simulink model "test_newfft_fun"  (Simulink 6.2)
settings: Solver=ode45  StartTime=0.0  StopTime=850  RelTol=1e-3
libraries: xbsIndex_r3 x554, simulink x1
(part 5 of 9)

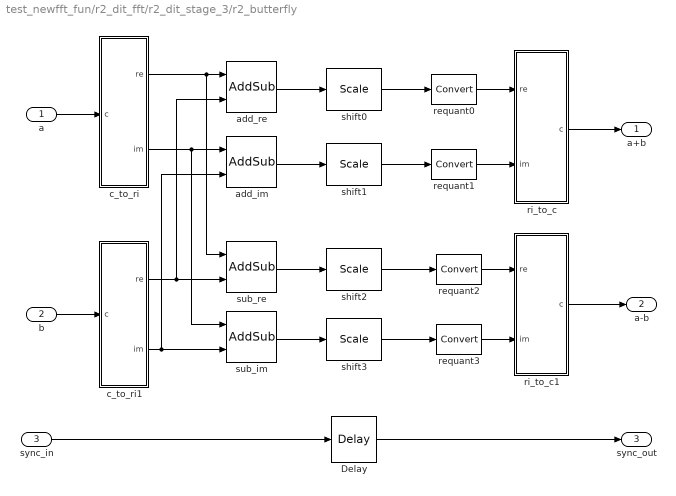
== system test_newfft_fun/r2_dit_fft/r2_dit_stage_3/r2_butterfly ==
  a : Inport  Port=1  LatchInput=off
  b : Inport  Port=2  LatchInput=off
  sync_in : Inport  Port=3  LatchInput=off
  Delay : xbsIndex_r3/Delay  latency=1  reg_retiming=off  explicit_period=off  period=1  en=off  accept_only_valid=off  init_zero=on  dbl_ovrd=off  show_param=off
      settings: xl_area=[0, 0, 0, 0, 0, 0, 0]
  add_im : xbsIndex_r3/AddSub  mode=Addition  precision=Full  arith_type=Unsigned  n_bits=8  bin_pt=2  quantization=Truncate  overflow=Wrap  latency=1  explicit_period=off  period=1  use_carryin=off  use_carryout=off  en=off  dbl_ovrd=off  show_param=on  use_core=on  pipeline=on  use_rpm=on  gen_core=off
      settings: xl_area=[0, 0, 0, 0, 0, 0, 0]
  add_re : xbsIndex_r3/AddSub  mode=Addition  precision=Full  arith_type=Unsigned  n_bits=8  bin_pt=2  quantization=Truncate  overflow=Wrap  latency=1  explicit_period=off  period=1  use_carryin=off  use_carryout=off  en=off  dbl_ovrd=off  show_param=on  use_core=on  pipeline=on  use_rpm=on  gen_core=off
      settings: xl_area=[0, 0, 0, 0, 0, 0, 0]
  c_to_ri : Subsystem  mask(Complex to Real-Imag){n_bits=10, bin_pt=0}
      mask prompts: n_bits "Bit Width"; bin_pt "Binary Point"
      mask help: Outputs real and imaginary components of a complex input.
      settings: AttributesFormatString=10_0 r/i
      mask Help:
      | <pre>
      | Description::
      | 
      | Outputs real and imaginary components of a complex input.
      | Useful for simplifying interconnects.
      | See also: Real-Imag to Complex (ri_to_c)
      | 
      | Mask Parameters::
      | 
      | Bit Width (n_bits): Specifies the width of the real/imaginary components.
      | Assumed equal for both components.
      | 
      | Binary Point (bin_pt): Specifies the binary point location in the real/imaginary components.
      | Assumed equal for both components.
      | </pre>
  c_to_ri1 : Subsystem  mask(Complex to Real-Imag){n_bits=10, bin_pt=0}
      mask prompts: n_bits "Bit Width"; bin_pt "Binary Point"
      mask help: Outputs real and imaginary components of a complex input.
      settings: AttributesFormatString=10_0 r/i
      mask Help:
      | <pre>
      | Description::
      | 
      | Outputs real and imaginary components of a complex input.
      | Useful for simplifying interconnects.
      | See also: Real-Imag to Complex (ri_to_c)
      | 
      | Mask Parameters::
      | 
      | Bit Width (n_bits): Specifies the width of the real/imaginary components.
      | Assumed equal for both components.
      | 
      | Binary Point (bin_pt): Specifies the binary point location in the real/imaginary components.
      | Assumed equal for both components.
      | </pre>
  requant{0..3} (4 alike) : xbsIndex_r3/Convert  arith_type="Signed  (2's comp)"  n_bits=11  bin_pt=0  quantization=Truncate  overflow=Wrap  latency=0  explicit_period=off  period=1  dbl_ovrd=off  show_param=on  inserted_by_tool=off  pipeline=on
      settings: xl_area=[0, 0, 0, 0, 0, 0, 0]
  ri_to_c : Subsystem
      mask Type: Real-Imag to Complex
      mask Description: Concatenates real and imaginary inputs into a complex output.
      mask Help:
      | <pre>
      | Description::
      | 
      | Concatenates a real and imaginary input into a complex output.
      | Useful for simplifying interconnects.
      | See also: Complex to Real-Imag (c_to_ri)
      | 
      | Mask Parameters::
      | 
      | (N/A)
      | </pre>
  ri_to_c1 : Subsystem
      mask Type: Real-Imag to Complex
      mask Description: Concatenates real and imaginary inputs into a complex output.
      mask Help:
      | <pre>
      | Description::
      | 
      | Concatenates a real and imaginary input into a complex output.
      | Useful for simplifying interconnects.
      | See also: Complex to Real-Imag (c_to_ri)
      | 
      | Mask Parameters::
      | 
      | (N/A)
      | </pre>
  shift{0..3} (4 alike) : xbsIndex_r3/Scale  scale_factor=0  explicit_period=off  period=1  dbl_ovrd=off
  sub_im : xbsIndex_r3/AddSub  mode=Subtraction  precision=Full  arith_type=Unsigned  n_bits=8  bin_pt=2  quantization=Truncate  overflow=Wrap  latency=1  explicit_period=off  period=1  use_carryin=off  use_carryout=off  en=off  dbl_ovrd=off  show_param=on  use_core=on  pipeline=on  use_rpm=on  gen_core=off
      settings: xl_area=[0, 0, 0, 0, 0, 0, 0]
  sub_re : xbsIndex_r3/AddSub  mode=Subtraction  precision=Full  arith_type=Unsigned  n_bits=8  bin_pt=2  quantization=Truncate  overflow=Wrap  latency=1  explicit_period=off  period=1  use_carryin=off  use_carryout=off  en=off  dbl_ovrd=off  show_param=on  use_core=on  pipeline=on  use_rpm=on  gen_core=off
      settings: xl_area=[0, 0, 0, 0, 0, 0, 0]
  a+b : Outport
  a-b : Outport  Port=2
  sync_out : Outport  Port=3
  wires:
  shift3/1 -> requant3/1
  sub_im/1 -> shift3/1
  shift2/1 -> requant2/1
  sub_re/1 -> shift2/1
  shift1/1 -> requant1/1
  shift0/1 -> requant0/1
  requant3/1 -> ri_to_c1/2(im)
  requant2/1 -> ri_to_c1/1(re)
  requant1/1 -> ri_to_c/2(im)
  requant0/1 -> ri_to_c/1(re)
  Delay/1 -> sync_out/1
  sync_in/1 -> Delay/1
  ri_to_c1/1(c) -> a-b/1
  ri_to_c/1(c) -> a+b/1
  add_im/1 -> shift1/1
  add_re/1 -> shift0/1
  a/1 -> c_to_ri/1(c)
  c_to_ri/2(im) -> sub_im/1, add_im/1
  c_to_ri/1(re) -> sub_re/1, add_re/1
  c_to_ri1/2(im) -> add_im/2, sub_im/2
  c_to_ri1/1(re) -> add_re/2, sub_re/2
  b/1 -> c_to_ri1/1(c)

== system test_newfft_fun/r2_dit_fft/r2_dit_stage_3/r2_twiddle ==
  a_in : Inport  Port=1  LatchInput=off
  b : Inport  Port=2  LatchInput=off
  sync_in : Inport  Port=3  LatchInput=off
  Delay1 : xbsIndex_r3/Delay  latency=1  reg_retiming=off  explicit_period=off  period=1  en=off  accept_only_valid=off  init_zero=on  dbl_ovrd=off  show_param=off
      settings: xl_area=[0, 0, 0, 0, 0, 0, 0]
  Delay2 : xbsIndex_r3/Delay  latency=1  reg_retiming=off  explicit_period=off  period=1  en=off  accept_only_valid=off  init_zero=on  dbl_ovrd=off  show_param=off
      settings: xl_area=[0, 0, 0, 0, 0, 0, 0]
  Delay3 : xbsIndex_r3/Delay  latency=1  reg_retiming=off  explicit_period=off  period=1  en=off  accept_only_valid=off  init_zero=on  dbl_ovrd=off  show_param=off
      settings: xl_area=[0, 0, 0, 0, 0, 0, 0]
  cmpy1 : Subsystem  mask(Complex Multiplier (4 real multipliers)){n_bits_b=10, bin_pt_b=9, n_bits_w=8, bin_pt_w=6, n_bits_bw=10, bin_pt_bw=9, quantization=Round  (unbiased: Even Values), overflow=Wrap, mult_latency=3, add_latency=1}
      mask prompts: n_bits_b "Number of Bits B"; bin_pt_b "Binary Point B"; n_bits_w "Number of Bits W"; bin_pt_w "Binary Point W"; n_bits_bw "Number of Bits BW"; bin_pt_bw "Binary Point BW"; mult_latency "Multiplier Latency"; add_latency "Adder Latency"
      mask help: This block multiplies two complex numbers using 4 real multipliers and 2 real adders. Pass-through paths are provided for another complex number and a sync signal. These pass through paths provide delay that matches the latency of the complex multiply operation.
      settings: AttributesFormatString=|
      | 10_9 * 8_6 ==> 10_9
      | round even, wrap
      | 3 mults
      mask Help:
      | <pre>
      | Description::
      | 
      | This block multiplies two complex numbers using 4 real multipliers and 2 real adders.
      | Pass-through paths are provided for another complex number and a sync signal.
      | These paths provide delay that matches the latency of the complex multiply operation.
      | 
      | a_in is passed through to a_out.
      | b and w complex inputs are multiplied and their product appears on the bw output.
      | sync_in is passed through to sync_out.
      | 
      | Mask Parameters::
      | 
      | Number of Bits B (n_bits_b): Specifies the width of the real/imaginary
      | components of input b.  Assumed equal for both components.
      | 
      | Binary Point B (bin_pt_b): Specifies the binary point point position of the
      | real/imaginary components of input b.  Assumed equal for both components.
      | 
      | Number of Bits W (n_bits_w): Specifies the width of the real/imaginary
      | components of input w.  Assumed equal for both components.
      | 
      | Binary Point W (bin_pt_w): Specifies the binary point point position of the
      | real/imaginary components of input w.  Assumed equal for both components.
      | 
      | Number of Bits BW (n_bits_bw): Specifies the width of the real/imaginary
      | components of output bw.  Assumed equal for both components.
      | 
      | Binary Point BW (bin_pt_bw): Specifies the binary point point position of the
      | real/imaginary components of output bw.  Assumed equal for both components.
      | 
      | Quantization (quantization): Specifies quantization handling.
      | 
      | Overflow (overflow): Specifies overflow handling.
      | 
      | Multiplier Latency (mult_latency): Latency to use for the underlying real multipliers.
      | 
      | Adder Latency (add_latency): Latency to use for the underlying real adders.
      | </pre>
      mask StyleString: edit,edit,edit,edit,edit,edit,popup(Truncate|Round  (unbiased: +/- Inf)|Round  (unbiased: Even Values)),popup(Wrap|Saturate|Error),edit,edit
  twiddle_gen1 : Subsystem  mask(Radix-R Twiddle Coefficient Generator (complex storage)){n_stages=8, radix=2, cur_stage=3, branch=1, decimation=Time, n_bits_w=8, bin_pt_w=6, use_bram=off}
      mask prompts: n_stages "Total Stages"; cur_stage "Current Stage"; decimation "Decimation Mode"; n_bits_w "Number of Bits"; bin_pt_w "Binary Point"; use_bram "Use BRAM"
      mask help: A radix-R twiddle coefficient generator using complex storage. Generates twiddle factors for Decimation in Time (i.e. twiddles before butterflies) or Decimation in Frequency (i.e. twiddles after butterflies) Fast Fourier Transforms of arbitrary-but-fixed radix. Radix must be a power of 2. Regardless of the decimation mode, the FFT is assumed to have inputs in normal order and outputs in bit-reversed order.
      settings: AttributesFormatString=|
      | depth 4
      | twiddle dist
      mask Help:
      | <pre>
      | Description::
      | 
      | A radix-R twiddle coefficient generator using complex storage.
      | 
      | Generates twiddle factors for Decimation in Time (i.e. twiddles before butterflies)
      | or Decimation in Frequency (i.e. twiddles after butterflies) Fast Fourier Transforms
      | of arbitrary-but-fixed radix.  Radix must be a power of 2.
      | 
      | Regardless of the decimation mode, the FFT is assumed to have inputs normally
      | ordered and outputs in bit-reversed order.
      | 
      | Complex storage means that the real and imaginary components are stored in
      | the same memory element.  This is generally fine, but if the combined width of
      | the real and imaginary components is greater than 18 and BRAM is being used
      | for the underlying storage, then the multiplier(s) adjacent to the BRAM(s) will
      | not be usable.  If that is a problem for your design, consider using the
      | "Radix-R Twiddle Coefficient Generator (real/imag storage)" block.
      | 
      | Mask Parameters::
      | 
      | Total Stages (n_stages):  The number of total stages in the FFT.
      | 
      | Radix (radix): The radix of the FFT.  The FFT will have radix^n_stages points.
      | 
      | Current Stage (cur_stage):  The number of the current stage for which this block should
      | generate twiddle coefficients.  Valid values are 3 through n_stages, inclusive.  Note that
      | stages are counted from 1 to n_stages for DIT (i.e. cur_stage==1 for the first stage) and
      | n_stages to 1 for DIF (i.e. cur_stage==1 for the last stage).
      | 
      | Branch (branch): The butterfly branch associated with this twiddle generator.
      | Valid values are 1 through radix-1, inclusive.
      | 
      | Decimation Mode (decimation): The decimation mode of the FFT.
      | 
      | Number of Bits (n_bits_w): Specifies the width of the real/imaginary components.
      | Assumed equal for both components.  This block outputs UFix_(2*n_bits_w)_0.
      | 
      | Use BRAM (use_bram): Check this checkbox to store twiddle coefficients in BRAM.
      | If unchecked, the coefficients will be sored in distributed memory (i.e. slices).
      | </pre>
      mask StyleString: edit,edit,edit,edit,popup(Time|Frequency),edit,edit,checkbox
  a_out : Outport
  bw : Outport  Port=2
  sync_out : Outport  Port=3
  wires:
  Delay3/1 -> cmpy1/4(sync_in)
  cmpy1/3(sync_out) -> sync_out/1
  twiddle_gen1/1(w) -> cmpy1/3(w)
  cmpy1/2(bw) -> bw/1
  Delay1/1 -> cmpy1/2(b)
  cmpy1/1(a_out) -> a_out/1
  Delay2/1 -> cmpy1/1(a_in)
  a_in/1 -> Delay2/1
  b/1 -> Delay1/1
  sync_in/1 -> Delay3/1, twiddle_gen1/1(sync_in)

== system test_newfft_fun/r2_dit_fft/r2_dit_stage_4/biplex_commutator ==
  AloAhi : Inport  Port=1  LatchInput=off
  BloBhi : Inport  Port=2  LatchInput=off
  sync_in : Inport  Port=3  LatchInput=off
  Counter : xbsIndex_r3/Counter  cnt_type=Free Running  n_bits=5  bin_pt=0  arith_type=Unsigned  start_count=0  cnt_to=Inf  cnt_by_val=1  operation=Up  explicit_period=off  period=1  load_pin=off  rst=on  en=off  dbl_ovrd=off  show_param=off  use_rpm=on  gen_core=off
      settings: xl_area=[0, 0, 0, 0, 0, 0, 0]
  Delay : xbsIndex_r3/Delay  latency=17  reg_retiming=off  explicit_period=off  period=1  en=off  accept_only_valid=off  init_zero=on  dbl_ovrd=off  show_param=off
      settings: xl_area=[0, 0, 0, 0, 0, 0, 0]
  Mux : xbsIndex_r3/Mux  inputs=2  precision=Full  arith_type="Signed  (2's comp)"  n_bits=8  bin_pt=2  quantization=Truncate  overflow=Wrap  latency=1  explicit_period=off  period=1  en=off  dbl_ovrd=off  show_param=off  mux_type=off  use_rpm=off  gen_core=off
      settings: xl_area=[0, 0, 0, 0, 0, 0, 0]
  Mux1 : xbsIndex_r3/Mux  inputs=2  precision=Full  arith_type="Signed  (2's comp)"  n_bits=8  bin_pt=2  quantization=Truncate  overflow=Wrap  latency=1  explicit_period=off  period=1  en=off  dbl_ovrd=off  show_param=on  mux_type=off  use_rpm=off  gen_core=off
      settings: xl_area=[0, 0, 0, 0, 0, 0, 0]
  delay_b : Subsystem  mask(SLR16 Delay){delay_depth=16}
      mask prompts: delay_depth "Delay Depth"
      mask help: A delay block that uses SLR16 elements for its storage.
      settings: AttributesFormatString=slr depth = 16
      mask Help:
      | <pre>
      | Description::
      | 
      | A delay block that uses SLR16 elements for its storage.
      | 
      | Mask Parameters::
      | 
      | Delay Depth (delay_depth): The length of the delay.
      | </pre>
  delay_lo : Subsystem  mask(SLR16 Delay){delay_depth=16}
      mask prompts: delay_depth "Delay Depth"
      mask help: A delay block that uses SLR16 elements for its storage.
      settings: AttributesFormatString=slr depth = 16
      mask Help:
      | <pre>
      | Description::
      | 
      | A delay block that uses SLR16 elements for its storage.
      | 
      | Mask Parameters::
      | 
      | Delay Depth (delay_depth): The length of the delay.
      | </pre>
  top_bit : xbsIndex_r3/Slice  mode=Upper Bit Location + Width  nbits=1  bit1=0  base1=MSB of Input  bit0=0  base0=LSB of Input  boolean_output=off  explicit_period=off  period=1  dbl_ovrd=off
  AloBlo : Outport
  AhiBhi : Outport  Port=2
  sync_out : Outport  Port=3
  wires:
  Delay/1 -> sync_out/1
  delay_lo/1(out) -> AloBlo/1
  Mux/1 -> delay_lo/1(in)
  delay_b/1(out) -> Mux/3, Mux1/2
  BloBhi/1 -> delay_b/1(in)
  Mux1/1 -> AhiBhi/1
  AloAhi/1 -> Mux1/3, Mux/2
  top_bit/1 -> Mux/1, Mux1/1
  Counter/1 -> top_bit/1
  sync_in/1 -> Delay/1, Counter/1

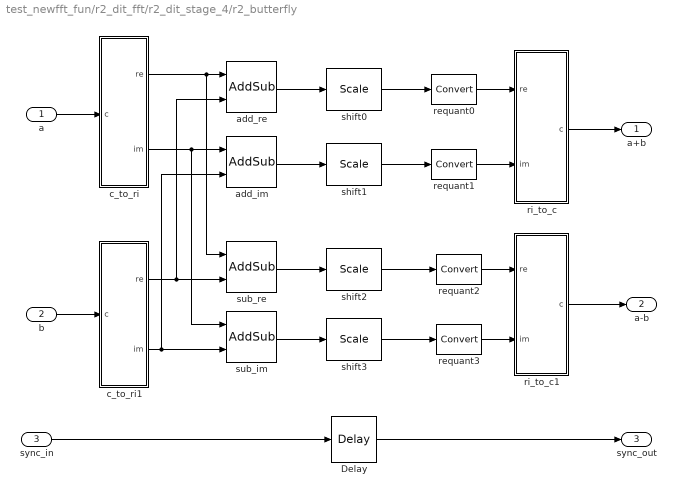
== system test_newfft_fun/r2_dit_fft/r2_dit_stage_4/r2_butterfly ==
  a : Inport  Port=1  LatchInput=off
  b : Inport  Port=2  LatchInput=off
  sync_in : Inport  Port=3  LatchInput=off
  Delay : xbsIndex_r3/Delay  latency=1  reg_retiming=off  explicit_period=off  period=1  en=off  accept_only_valid=off  init_zero=on  dbl_ovrd=off  show_param=off
      settings: xl_area=[0, 0, 0, 0, 0, 0, 0]
  add_im : xbsIndex_r3/AddSub  mode=Addition  precision=Full  arith_type=Unsigned  n_bits=8  bin_pt=2  quantization=Truncate  overflow=Wrap  latency=1  explicit_period=off  period=1  use_carryin=off  use_carryout=off  en=off  dbl_ovrd=off  show_param=on  use_core=on  pipeline=on  use_rpm=on  gen_core=off
      settings: xl_area=[0, 0, 0, 0, 0, 0, 0]
  add_re : xbsIndex_r3/AddSub  mode=Addition  precision=Full  arith_type=Unsigned  n_bits=8  bin_pt=2  quantization=Truncate  overflow=Wrap  latency=1  explicit_period=off  period=1  use_carryin=off  use_carryout=off  en=off  dbl_ovrd=off  show_param=on  use_core=on  pipeline=on  use_rpm=on  gen_core=off
      settings: xl_area=[0, 0, 0, 0, 0, 0, 0]
  c_to_ri : Subsystem  mask(Complex to Real-Imag){n_bits=11, bin_pt=0}
      mask prompts: n_bits "Bit Width"; bin_pt "Binary Point"
      mask help: Outputs real and imaginary components of a complex input.
      settings: AttributesFormatString=11_0 r/i
      mask Help:
      | <pre>
      | Description::
      | 
      | Outputs real and imaginary components of a complex input.
      | Useful for simplifying interconnects.
      | See also: Real-Imag to Complex (ri_to_c)
      | 
      | Mask Parameters::
      | 
      | Bit Width (n_bits): Specifies the width of the real/imaginary components.
      | Assumed equal for both components.
      | 
      | Binary Point (bin_pt): Specifies the binary point location in the real/imaginary components.
      | Assumed equal for both components.
      | </pre>
  c_to_ri1 : Subsystem  mask(Complex to Real-Imag){n_bits=11, bin_pt=0}
      mask prompts: n_bits "Bit Width"; bin_pt "Binary Point"
      mask help: Outputs real and imaginary components of a complex input.
      settings: AttributesFormatString=11_0 r/i
      mask Help:
      | <pre>
      | Description::
      | 
      | Outputs real and imaginary components of a complex input.
      | Useful for simplifying interconnects.
      | See also: Real-Imag to Complex (ri_to_c)
      | 
      | Mask Parameters::
      | 
      | Bit Width (n_bits): Specifies the width of the real/imaginary components.
      | Assumed equal for both components.
      | 
      | Binary Point (bin_pt): Specifies the binary point location in the real/imaginary components.
      | Assumed equal for both components.
      | </pre>
  requant{0..3} (4 alike) : xbsIndex_r3/Convert  arith_type="Signed  (2's comp)"  n_bits=12  bin_pt=0  quantization=Truncate  overflow=Wrap  latency=0  explicit_period=off  period=1  dbl_ovrd=off  show_param=on  inserted_by_tool=off  pipeline=on
      settings: xl_area=[0, 0, 0, 0, 0, 0, 0]
  ri_to_c : Subsystem
      mask Type: Real-Imag to Complex
      mask Description: Concatenates real and imaginary inputs into a complex output.
      mask Help:
      | <pre>
      | Description::
      | 
      | Concatenates a real and imaginary input into a complex output.
      | Useful for simplifying interconnects.
      | See also: Complex to Real-Imag (c_to_ri)
      | 
      | Mask Parameters::
      | 
      | (N/A)
      | </pre>
  ri_to_c1 : Subsystem
      mask Type: Real-Imag to Complex
      mask Description: Concatenates real and imaginary inputs into a complex output.
      mask Help:
      | <pre>
      | Description::
      | 
      | Concatenates a real and imaginary input into a complex output.
      | Useful for simplifying interconnects.
      | See also: Complex to Real-Imag (c_to_ri)
      | 
      | Mask Parameters::
      | 
      | (N/A)
      | </pre>
  shift{0..3} (4 alike) : xbsIndex_r3/Scale  scale_factor=0  explicit_period=off  period=1  dbl_ovrd=off
  sub_im : xbsIndex_r3/AddSub  mode=Subtraction  precision=Full  arith_type=Unsigned  n_bits=8  bin_pt=2  quantization=Truncate  overflow=Wrap  latency=1  explicit_period=off  period=1  use_carryin=off  use_carryout=off  en=off  dbl_ovrd=off  show_param=on  use_core=on  pipeline=on  use_rpm=on  gen_core=off
      settings: xl_area=[0, 0, 0, 0, 0, 0, 0]
  sub_re : xbsIndex_r3/AddSub  mode=Subtraction  precision=Full  arith_type=Unsigned  n_bits=8  bin_pt=2  quantization=Truncate  overflow=Wrap  latency=1  explicit_period=off  period=1  use_carryin=off  use_carryout=off  en=off  dbl_ovrd=off  show_param=on  use_core=on  pipeline=on  use_rpm=on  gen_core=off
      settings: xl_area=[0, 0, 0, 0, 0, 0, 0]
  a+b : Outport
  a-b : Outport  Port=2
  sync_out : Outport  Port=3
  wires:
  shift3/1 -> requant3/1
  sub_im/1 -> shift3/1
  shift2/1 -> requant2/1
  sub_re/1 -> shift2/1
  shift1/1 -> requant1/1
  shift0/1 -> requant0/1
  requant3/1 -> ri_to_c1/2(im)
  requant2/1 -> ri_to_c1/1(re)
  requant1/1 -> ri_to_c/2(im)
  requant0/1 -> ri_to_c/1(re)
  Delay/1 -> sync_out/1
  sync_in/1 -> Delay/1
  ri_to_c1/1(c) -> a-b/1
  ri_to_c/1(c) -> a+b/1
  add_im/1 -> shift1/1
  add_re/1 -> shift0/1
  a/1 -> c_to_ri/1(c)
  c_to_ri/2(im) -> sub_im/1, add_im/1
  c_to_ri/1(re) -> sub_re/1, add_re/1
  c_to_ri1/2(im) -> add_im/2, sub_im/2
  c_to_ri1/1(re) -> add_re/2, sub_re/2
  b/1 -> c_to_ri1/1(c)

== system test_newfft_fun/r2_dit_fft/r2_dit_stage_4/r2_twiddle ==
  a_in : Inport  Port=1  LatchInput=off
  b : Inport  Port=2  LatchInput=off
  sync_in : Inport  Port=3  LatchInput=off
  Delay1 : xbsIndex_r3/Delay  latency=1  reg_retiming=off  explicit_period=off  period=1  en=off  accept_only_valid=off  init_zero=on  dbl_ovrd=off  show_param=off
      settings: xl_area=[0, 0, 0, 0, 0, 0, 0]
  Delay2 : xbsIndex_r3/Delay  latency=1  reg_retiming=off  explicit_period=off  period=1  en=off  accept_only_valid=off  init_zero=on  dbl_ovrd=off  show_param=off
      settings: xl_area=[0, 0, 0, 0, 0, 0, 0]
  Delay3 : xbsIndex_r3/Delay  latency=1  reg_retiming=off  explicit_period=off  period=1  en=off  accept_only_valid=off  init_zero=on  dbl_ovrd=off  show_param=off
      settings: xl_area=[0, 0, 0, 0, 0, 0, 0]
  cmpy1 : Subsystem  mask(Complex Multiplier (4 real multipliers)){n_bits_b=11, bin_pt_b=10, n_bits_w=8, bin_pt_w=6, n_bits_bw=11, bin_pt_bw=10, quantization=Round  (unbiased: Even Values), overflow=Wrap, mult_latency=3, add_latency=1}
      mask prompts: n_bits_b "Number of Bits B"; bin_pt_b "Binary Point B"; n_bits_w "Number of Bits W"; bin_pt_w "Binary Point W"; n_bits_bw "Number of Bits BW"; bin_pt_bw "Binary Point BW"; mult_latency "Multiplier Latency"; add_latency "Adder Latency"
      mask help: This block multiplies two complex numbers using 4 real multipliers and 2 real adders. Pass-through paths are provided for another complex number and a sync signal. These pass through paths provide delay that matches the latency of the complex multiply operation.
      settings: AttributesFormatString=|
      | 11_10 * 8_6 ==> 11_10
      | round even, wrap
      | 3 mults
      mask Help:
      | <pre>
      | Description::
      | 
      | This block multiplies two complex numbers using 4 real multipliers and 2 real adders.
      | Pass-through paths are provided for another complex number and a sync signal.
      | These paths provide delay that matches the latency of the complex multiply operation.
      | 
      | a_in is passed through to a_out.
      | b and w complex inputs are multiplied and their product appears on the bw output.
      | sync_in is passed through to sync_out.
      | 
      | Mask Parameters::
      | 
      | Number of Bits B (n_bits_b): Specifies the width of the real/imaginary
      | components of input b.  Assumed equal for both components.
      | 
      | Binary Point B (bin_pt_b): Specifies the binary point point position of the
      | real/imaginary components of input b.  Assumed equal for both components.
      | 
      | Number of Bits W (n_bits_w): Specifies the width of the real/imaginary
      | components of input w.  Assumed equal for both components.
      | 
      | Binary Point W (bin_pt_w): Specifies the binary point point position of the
      | real/imaginary components of input w.  Assumed equal for both components.
      | 
      | Number of Bits BW (n_bits_bw): Specifies the width of the real/imaginary
      | components of output bw.  Assumed equal for both components.
      | 
      | Binary Point BW (bin_pt_bw): Specifies the binary point point position of the
      | real/imaginary components of output bw.  Assumed equal for both components.
      | 
      | Quantization (quantization): Specifies quantization handling.
      | 
      | Overflow (overflow): Specifies overflow handling.
      | 
      | Multiplier Latency (mult_latency): Latency to use for the underlying real multipliers.
      | 
      | Adder Latency (add_latency): Latency to use for the underlying real adders.
      | </pre>
      mask StyleString: edit,edit,edit,edit,edit,edit,popup(Truncate|Round  (unbiased: +/- Inf)|Round  (unbiased: Even Values)),popup(Wrap|Saturate|Error),edit,edit
  twiddle_gen1 : Subsystem  mask(Radix-R Twiddle Coefficient Generator (complex storage)){n_stages=8, radix=2, cur_stage=4, branch=1, decimation=Time, n_bits_w=8, bin_pt_w=6, use_bram=off}
      mask prompts: n_stages "Total Stages"; cur_stage "Current Stage"; decimation "Decimation Mode"; n_bits_w "Number of Bits"; bin_pt_w "Binary Point"; use_bram "Use BRAM"
      mask help: A radix-R twiddle coefficient generator using complex storage. Generates twiddle factors for Decimation in Time (i.e. twiddles before butterflies) or Decimation in Frequency (i.e. twiddles after butterflies) Fast Fourier Transforms of arbitrary-but-fixed radix. Radix must be a power of 2. Regardless of the decimation mode, the FFT is assumed to have inputs in normal order and outputs in bit-reversed order.
      settings: AttributesFormatString=|
      | depth 8
      | twiddle dist
      mask Help:
      | <pre>
      | Description::
      | 
      | A radix-R twiddle coefficient generator using complex storage.
      | 
      | Generates twiddle factors for Decimation in Time (i.e. twiddles before butterflies)
      | or Decimation in Frequency (i.e. twiddles after butterflies) Fast Fourier Transforms
      | of arbitrary-but-fixed radix.  Radix must be a power of 2.
      | 
      | Regardless of the decimation mode, the FFT is assumed to have inputs normally
      | ordered and outputs in bit-reversed order.
      | 
      | Complex storage means that the real and imaginary components are stored in
      | the same memory element.  This is generally fine, but if the combined width of
      | the real and imaginary components is greater than 18 and BRAM is being used
      | for the underlying storage, then the multiplier(s) adjacent to the BRAM(s) will
      | not be usable.  If that is a problem for your design, consider using the
      | "Radix-R Twiddle Coefficient Generator (real/imag storage)" block.
      | 
      | Mask Parameters::
      | 
      | Total Stages (n_stages):  The number of total stages in the FFT.
      | 
      | Radix (radix): The radix of the FFT.  The FFT will have radix^n_stages points.
      | 
      | Current Stage (cur_stage):  The number of the current stage for which this block should
      | generate twiddle coefficients.  Valid values are 3 through n_stages, inclusive.  Note that
      | stages are counted from 1 to n_stages for DIT (i.e. cur_stage==1 for the first stage) and
      | n_stages to 1 for DIF (i.e. cur_stage==1 for the last stage).
      | 
      | Branch (branch): The butterfly branch associated with this twiddle generator.
      | Valid values are 1 through radix-1, inclusive.
      | 
      | Decimation Mode (decimation): The decimation mode of the FFT.
      | 
      | Number of Bits (n_bits_w): Specifies the width of the real/imaginary components.
      | Assumed equal for both components.  This block outputs UFix_(2*n_bits_w)_0.
      | 
      | Use BRAM (use_bram): Check this checkbox to store twiddle coefficients in BRAM.
      | If unchecked, the coefficients will be sored in distributed memory (i.e. slices).
      | </pre>
      mask StyleString: edit,edit,edit,edit,popup(Time|Frequency),edit,edit,checkbox
  a_out : Outport
  bw : Outport  Port=2
  sync_out : Outport  Port=3
  wires:
  Delay3/1 -> cmpy1/4(sync_in)
  cmpy1/3(sync_out) -> sync_out/1
  twiddle_gen1/1(w) -> cmpy1/3(w)
  cmpy1/2(bw) -> bw/1
  Delay1/1 -> cmpy1/2(b)
  cmpy1/1(a_out) -> a_out/1
  Delay2/1 -> cmpy1/1(a_in)
  a_in/1 -> Delay2/1
  b/1 -> Delay1/1
  sync_in/1 -> Delay3/1, twiddle_gen1/1(sync_in)

== system test_newfft_fun/r2_dit_fft/r2_dit_stage_5/biplex_commutator ==
  AloAhi : Inport  Port=1  LatchInput=off
  BloBhi : Inport  Port=2  LatchInput=off
  sync_in : Inport  Port=3  LatchInput=off
  Counter : xbsIndex_r3/Counter  cnt_type=Free Running  n_bits=4  bin_pt=0  arith_type=Unsigned  start_count=0  cnt_to=Inf  cnt_by_val=1  operation=Up  explicit_period=off  period=1  load_pin=off  rst=on  en=off  dbl_ovrd=off  show_param=off  use_rpm=on  gen_core=off
      settings: xl_area=[0, 0, 0, 0, 0, 0, 0]
  Delay : xbsIndex_r3/Delay  latency=9  reg_retiming=off  explicit_period=off  period=1  en=off  accept_only_valid=off  init_zero=on  dbl_ovrd=off  show_param=off
      settings: xl_area=[0, 0, 0, 0, 0, 0, 0]
  Mux : xbsIndex_r3/Mux  inputs=2  precision=Full  arith_type="Signed  (2's comp)"  n_bits=8  bin_pt=2  quantization=Truncate  overflow=Wrap  latency=1  explicit_period=off  period=1  en=off  dbl_ovrd=off  show_param=off  mux_type=off  use_rpm=off  gen_core=off
      settings: xl_area=[0, 0, 0, 0, 0, 0, 0]
  Mux1 : xbsIndex_r3/Mux  inputs=2  precision=Full  arith_type="Signed  (2's comp)"  n_bits=8  bin_pt=2  quantization=Truncate  overflow=Wrap  latency=1  explicit_period=off  period=1  en=off  dbl_ovrd=off  show_param=on  mux_type=off  use_rpm=off  gen_core=off
      settings: xl_area=[0, 0, 0, 0, 0, 0, 0]
  delay_b : Subsystem  mask(SLR16 Delay){delay_depth=8}
      mask prompts: delay_depth "Delay Depth"
      mask help: A delay block that uses SLR16 elements for its storage.
      settings: AttributesFormatString=slr depth = 8
      mask Help:
      | <pre>
      | Description::
      | 
      | A delay block that uses SLR16 elements for its storage.
      | 
      | Mask Parameters::
      | 
      | Delay Depth (delay_depth): The length of the delay.
      | </pre>
  delay_lo : Subsystem  mask(SLR16 Delay){delay_depth=8}
      mask prompts: delay_depth "Delay Depth"
      mask help: A delay block that uses SLR16 elements for its storage.
      settings: AttributesFormatString=slr depth = 8
      mask Help:
      | <pre>
      | Description::
      | 
      | A delay block that uses SLR16 elements for its storage.
      | 
      | Mask Parameters::
      | 
      | Delay Depth (delay_depth): The length of the delay.
      | </pre>
  top_bit : xbsIndex_r3/Slice  mode=Upper Bit Location + Width  nbits=1  bit1=0  base1=MSB of Input  bit0=0  base0=LSB of Input  boolean_output=off  explicit_period=off  period=1  dbl_ovrd=off
  AloBlo : Outport
  AhiBhi : Outport  Port=2
  sync_out : Outport  Port=3
  wires:
  Delay/1 -> sync_out/1
  delay_lo/1(out) -> AloBlo/1
  Mux/1 -> delay_lo/1(in)
  delay_b/1(out) -> Mux/3, Mux1/2
  BloBhi/1 -> delay_b/1(in)
  Mux1/1 -> AhiBhi/1
  AloAhi/1 -> Mux1/3, Mux/2
  top_bit/1 -> Mux/1, Mux1/1
  Counter/1 -> top_bit/1
  sync_in/1 -> Delay/1, Counter/1

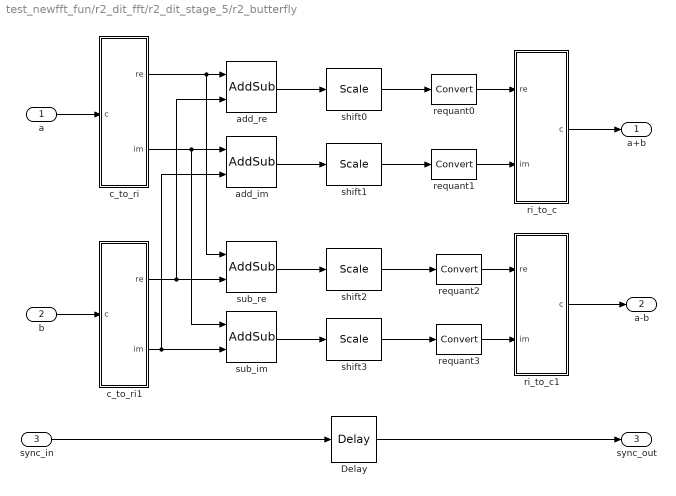
== system test_newfft_fun/r2_dit_fft/r2_dit_stage_5/r2_butterfly ==
  a : Inport  Port=1  LatchInput=off
  b : Inport  Port=2  LatchInput=off
  sync_in : Inport  Port=3  LatchInput=off
  Delay : xbsIndex_r3/Delay  latency=1  reg_retiming=off  explicit_period=off  period=1  en=off  accept_only_valid=off  init_zero=on  dbl_ovrd=off  show_param=off
      settings: xl_area=[0, 0, 0, 0, 0, 0, 0]
  add_im : xbsIndex_r3/AddSub  mode=Addition  precision=Full  arith_type=Unsigned  n_bits=8  bin_pt=2  quantization=Truncate  overflow=Wrap  latency=1  explicit_period=off  period=1  use_carryin=off  use_carryout=off  en=off  dbl_ovrd=off  show_param=on  use_core=on  pipeline=on  use_rpm=on  gen_core=off
      settings: xl_area=[0, 0, 0, 0, 0, 0, 0]
  add_re : xbsIndex_r3/AddSub  mode=Addition  precision=Full  arith_type=Unsigned  n_bits=8  bin_pt=2  quantization=Truncate  overflow=Wrap  latency=1  explicit_period=off  period=1  use_carryin=off  use_carryout=off  en=off  dbl_ovrd=off  show_param=on  use_core=on  pipeline=on  use_rpm=on  gen_core=off
      settings: xl_area=[0, 0, 0, 0, 0, 0, 0]
  c_to_ri : Subsystem  mask(Complex to Real-Imag){n_bits=12, bin_pt=0}
      mask prompts: n_bits "Bit Width"; bin_pt "Binary Point"
      mask help: Outputs real and imaginary components of a complex input.
      settings: AttributesFormatString=12_0 r/i
      mask Help:
      | <pre>
      | Description::
      | 
      | Outputs real and imaginary components of a complex input.
      | Useful for simplifying interconnects.
      | See also: Real-Imag to Complex (ri_to_c)
      | 
      | Mask Parameters::
      | 
      | Bit Width (n_bits): Specifies the width of the real/imaginary components.
      | Assumed equal for both components.
      | 
      | Binary Point (bin_pt): Specifies the binary point location in the real/imaginary components.
      | Assumed equal for both components.
      | </pre>
  c_to_ri1 : Subsystem  mask(Complex to Real-Imag){n_bits=12, bin_pt=0}
      mask prompts: n_bits "Bit Width"; bin_pt "Binary Point"
      mask help: Outputs real and imaginary components of a complex input.
      settings: AttributesFormatString=12_0 r/i
      mask Help:
      | <pre>
      | Description::
      | 
      | Outputs real and imaginary components of a complex input.
      | Useful for simplifying interconnects.
      | See also: Real-Imag to Complex (ri_to_c)
      | 
      | Mask Parameters::
      | 
      | Bit Width (n_bits): Specifies the width of the real/imaginary components.
      | Assumed equal for both components.
      | 
      | Binary Point (bin_pt): Specifies the binary point location in the real/imaginary components.
      | Assumed equal for both components.
      | </pre>
  requant{0..3} (4 alike) : xbsIndex_r3/Convert  arith_type="Signed  (2's comp)"  n_bits=13  bin_pt=0  quantization=Truncate  overflow=Wrap  latency=0  explicit_period=off  period=1  dbl_ovrd=off  show_param=on  inserted_by_tool=off  pipeline=on
      settings: xl_area=[0, 0, 0, 0, 0, 0, 0]
  ri_to_c : Subsystem
      mask Type: Real-Imag to Complex
      mask Description: Concatenates real and imaginary inputs into a complex output.
      mask Help:
      | <pre>
      | Description::
      | 
      | Concatenates a real and imaginary input into a complex output.
      | Useful for simplifying interconnects.
      | See also: Complex to Real-Imag (c_to_ri)
      | 
      | Mask Parameters::
      | 
      | (N/A)
      | </pre>
  ri_to_c1 : Subsystem
      mask Type: Real-Imag to Complex
      mask Description: Concatenates real and imaginary inputs into a complex output.
      mask Help:
      | <pre>
      | Description::
      | 
      | Concatenates a real and imaginary input into a complex output.
      | Useful for simplifying interconnects.
      | See also: Complex to Real-Imag (c_to_ri)
      | 
      | Mask Parameters::
      | 
      | (N/A)
      | </pre>
  shift{0..3} (4 alike) : xbsIndex_r3/Scale  scale_factor=0  explicit_period=off  period=1  dbl_ovrd=off
  sub_im : xbsIndex_r3/AddSub  mode=Subtraction  precision=Full  arith_type=Unsigned  n_bits=8  bin_pt=2  quantization=Truncate  overflow=Wrap  latency=1  explicit_period=off  period=1  use_carryin=off  use_carryout=off  en=off  dbl_ovrd=off  show_param=on  use_core=on  pipeline=on  use_rpm=on  gen_core=off
      settings: xl_area=[0, 0, 0, 0, 0, 0, 0]
  sub_re : xbsIndex_r3/AddSub  mode=Subtraction  precision=Full  arith_type=Unsigned  n_bits=8  bin_pt=2  quantization=Truncate  overflow=Wrap  latency=1  explicit_period=off  period=1  use_carryin=off  use_carryout=off  en=off  dbl_ovrd=off  show_param=on  use_core=on  pipeline=on  use_rpm=on  gen_core=off
      settings: xl_area=[0, 0, 0, 0, 0, 0, 0]
  a+b : Outport
  a-b : Outport  Port=2
  sync_out : Outport  Port=3
  wires:
  shift3/1 -> requant3/1
  sub_im/1 -> shift3/1
  shift2/1 -> requant2/1
  sub_re/1 -> shift2/1
  shift1/1 -> requant1/1
  shift0/1 -> requant0/1
  requant3/1 -> ri_to_c1/2(im)
  requant2/1 -> ri_to_c1/1(re)
  requant1/1 -> ri_to_c/2(im)
  requant0/1 -> ri_to_c/1(re)
  Delay/1 -> sync_out/1
  sync_in/1 -> Delay/1
  ri_to_c1/1(c) -> a-b/1
  ri_to_c/1(c) -> a+b/1
  add_im/1 -> shift1/1
  add_re/1 -> shift0/1
  a/1 -> c_to_ri/1(c)
  c_to_ri/2(im) -> sub_im/1, add_im/1
  c_to_ri/1(re) -> sub_re/1, add_re/1
  c_to_ri1/2(im) -> add_im/2, sub_im/2
  c_to_ri1/1(re) -> add_re/2, sub_re/2
  b/1 -> c_to_ri1/1(c)

== system test_newfft_fun/r2_dit_fft/r2_dit_stage_5/r2_twiddle ==
  a_in : Inport  Port=1  LatchInput=off
  b : Inport  Port=2  LatchInput=off
  sync_in : Inport  Port=3  LatchInput=off
  Delay1 : xbsIndex_r3/Delay  latency=1  reg_retiming=off  explicit_period=off  period=1  en=off  accept_only_valid=off  init_zero=on  dbl_ovrd=off  show_param=off
      settings: xl_area=[0, 0, 0, 0, 0, 0, 0]
  Delay2 : xbsIndex_r3/Delay  latency=1  reg_retiming=off  explicit_period=off  period=1  en=off  accept_only_valid=off  init_zero=on  dbl_ovrd=off  show_param=off
      settings: xl_area=[0, 0, 0, 0, 0, 0, 0]
  Delay3 : xbsIndex_r3/Delay  latency=1  reg_retiming=off  explicit_period=off  period=1  en=off  accept_only_valid=off  init_zero=on  dbl_ovrd=off  show_param=off
      settings: xl_area=[0, 0, 0, 0, 0, 0, 0]
  cmpy1 : Subsystem  mask(Complex Multiplier (4 real multipliers)){n_bits_b=12, bin_pt_b=11, n_bits_w=8, bin_pt_w=6, n_bits_bw=12, bin_pt_bw=11, quantization=Round  (unbiased: Even Values), overflow=Wrap, mult_latency=3, add_latency=1}
      mask prompts: n_bits_b "Number of Bits B"; bin_pt_b "Binary Point B"; n_bits_w "Number of Bits W"; bin_pt_w "Binary Point W"; n_bits_bw "Number of Bits BW"; bin_pt_bw "Binary Point BW"; mult_latency "Multiplier Latency"; add_latency "Adder Latency"
      mask help: This block multiplies two complex numbers using 4 real multipliers and 2 real adders. Pass-through paths are provided for another complex number and a sync signal. These pass through paths provide delay that matches the latency of the complex multiply operation.
      settings: AttributesFormatString=|
      | 12_11 * 8_6 ==> 12_11
      | round even, wrap
      | 3 mults
      mask Help:
      | <pre>
      | Description::
      | 
      | This block multiplies two complex numbers using 4 real multipliers and 2 real adders.
      | Pass-through paths are provided for another complex number and a sync signal.
      | These paths provide delay that matches the latency of the complex multiply operation.
      | 
      | a_in is passed through to a_out.
      | b and w complex inputs are multiplied and their product appears on the bw output.
      | sync_in is passed through to sync_out.
      | 
      | Mask Parameters::
      | 
      | Number of Bits B (n_bits_b): Specifies the width of the real/imaginary
      | components of input b.  Assumed equal for both components.
      | 
      | Binary Point B (bin_pt_b): Specifies the binary point point position of the
      | real/imaginary components of input b.  Assumed equal for both components.
      | 
      | Number of Bits W (n_bits_w): Specifies the width of the real/imaginary
      | components of input w.  Assumed equal for both components.
      | 
      | Binary Point W (bin_pt_w): Specifies the binary point point position of the
      | real/imaginary components of input w.  Assumed equal for both components.
      | 
      | Number of Bits BW (n_bits_bw): Specifies the width of the real/imaginary
      | components of output bw.  Assumed equal for both components.
      | 
      | Binary Point BW (bin_pt_bw): Specifies the binary point point position of the
      | real/imaginary components of output bw.  Assumed equal for both components.
      | 
      | Quantization (quantization): Specifies quantization handling.
      | 
      | Overflow (overflow): Specifies overflow handling.
      | 
      | Multiplier Latency (mult_latency): Latency to use for the underlying real multipliers.
      | 
      | Adder Latency (add_latency): Latency to use for the underlying real adders.
      | </pre>
      mask StyleString: edit,edit,edit,edit,edit,edit,popup(Truncate|Round  (unbiased: +/- Inf)|Round  (unbiased: Even Values)),popup(Wrap|Saturate|Error),edit,edit
  twiddle_gen1 : Subsystem  mask(Radix-R Twiddle Coefficient Generator (complex storage)){n_stages=8, radix=2, cur_stage=5, branch=1, decimation=Time, n_bits_w=8, bin_pt_w=6, use_bram=off}
      mask prompts: n_stages "Total Stages"; cur_stage "Current Stage"; decimation "Decimation Mode"; n_bits_w "Number of Bits"; bin_pt_w "Binary Point"; use_bram "Use BRAM"
      mask help: A radix-R twiddle coefficient generator using complex storage. Generates twiddle factors for Decimation in Time (i.e. twiddles before butterflies) or Decimation in Frequency (i.e. twiddles after butterflies) Fast Fourier Transforms of arbitrary-but-fixed radix. Radix must be a power of 2. Regardless of the decimation mode, the FFT is assumed to have inputs in normal order and outputs in bit-reversed order.
      settings: AttributesFormatString=|
      | depth 16
      | twiddle dist
      mask Help:
      | <pre>
      | Description::
      | 
      | A radix-R twiddle coefficient generator using complex storage.
      | 
      | Generates twiddle factors for Decimation in Time (i.e. twiddles before butterflies)
      | or Decimation in Frequency (i.e. twiddles after butterflies) Fast Fourier Transforms
      | of arbitrary-but-fixed radix.  Radix must be a power of 2.
      | 
      | Regardless of the decimation mode, the FFT is assumed to have inputs normally
      | ordered and outputs in bit-reversed order.
      | 
      | Complex storage means that the real and imaginary components are stored in
      | the same memory element.  This is generally fine, but if the combined width of
      | the real and imaginary components is greater than 18 and BRAM is being used
      | for the underlying storage, then the multiplier(s) adjacent to the BRAM(s) will
      | not be usable.  If that is a problem for your design, consider using the
      | "Radix-R Twiddle Coefficient Generator (real/imag storage)" block.
      | 
      | Mask Parameters::
      | 
      | Total Stages (n_stages):  The number of total stages in the FFT.
      | 
      | Radix (radix): The radix of the FFT.  The FFT will have radix^n_stages points.
      | 
      | Current Stage (cur_stage):  The number of the current stage for which this block should
      | generate twiddle coefficients.  Valid values are 3 through n_stages, inclusive.  Note that
      | stages are counted from 1 to n_stages for DIT (i.e. cur_stage==1 for the first stage) and
      | n_stages to 1 for DIF (i.e. cur_stage==1 for the last stage).
      | 
      | Branch (branch): The butterfly branch associated with this twiddle generator.
      | Valid values are 1 through radix-1, inclusive.
      | 
      | Decimation Mode (decimation): The decimation mode of the FFT.
      | 
      | Number of Bits (n_bits_w): Specifies the width of the real/imaginary components.
      | Assumed equal for both components.  This block outputs UFix_(2*n_bits_w)_0.
      | 
      | Use BRAM (use_bram): Check this checkbox to store twiddle coefficients in BRAM.
      | If unchecked, the coefficients will be sored in distributed memory (i.e. slices).
      | </pre>
      mask StyleString: edit,edit,edit,edit,popup(Time|Frequency),edit,edit,checkbox
  a_out : Outport
  bw : Outport  Port=2
  sync_out : Outport  Port=3
  wires:
  Delay3/1 -> cmpy1/4(sync_in)
  cmpy1/3(sync_out) -> sync_out/1
  twiddle_gen1/1(w) -> cmpy1/3(w)
  cmpy1/2(bw) -> bw/1
  Delay1/1 -> cmpy1/2(b)
  cmpy1/1(a_out) -> a_out/1
  Delay2/1 -> cmpy1/1(a_in)
  a_in/1 -> Delay2/1
  b/1 -> Delay1/1
  sync_in/1 -> Delay3/1, twiddle_gen1/1(sync_in)

== system test_newfft_fun/r2_dit_fft/r2_dit_stage_6/biplex_commutator ==
  AloAhi : Inport  Port=1  LatchInput=off
  BloBhi : Inport  Port=2  LatchInput=off
  sync_in : Inport  Port=3  LatchInput=off
  Counter : xbsIndex_r3/Counter  cnt_type=Free Running  n_bits=3  bin_pt=0  arith_type=Unsigned  start_count=0  cnt_to=Inf  cnt_by_val=1  operation=Up  explicit_period=off  period=1  load_pin=off  rst=on  en=off  dbl_ovrd=off  show_param=off  use_rpm=on  gen_core=off
      settings: xl_area=[0, 0, 0, 0, 0, 0, 0]
  Delay : xbsIndex_r3/Delay  latency=5  reg_retiming=off  explicit_period=off  period=1  en=off  accept_only_valid=off  init_zero=on  dbl_ovrd=off  show_param=off
      settings: xl_area=[0, 0, 0, 0, 0, 0, 0]
  Mux : xbsIndex_r3/Mux  inputs=2  precision=Full  arith_type="Signed  (2's comp)"  n_bits=8  bin_pt=2  quantization=Truncate  overflow=Wrap  latency=1  explicit_period=off  period=1  en=off  dbl_ovrd=off  show_param=off  mux_type=off  use_rpm=off  gen_core=off
      settings: xl_area=[0, 0, 0, 0, 0, 0, 0]
  Mux1 : xbsIndex_r3/Mux  inputs=2  precision=Full  arith_type="Signed  (2's comp)"  n_bits=8  bin_pt=2  quantization=Truncate  overflow=Wrap  latency=1  explicit_period=off  period=1  en=off  dbl_ovrd=off  show_param=on  mux_type=off  use_rpm=off  gen_core=off
      settings: xl_area=[0, 0, 0, 0, 0, 0, 0]
  delay_b : Subsystem  mask(SLR16 Delay){delay_depth=4}
      mask prompts: delay_depth "Delay Depth"
      mask help: A delay block that uses SLR16 elements for its storage.
      settings: AttributesFormatString=slr depth = 4
      mask Help:
      | <pre>
      | Description::
      | 
      | A delay block that uses SLR16 elements for its storage.
      | 
      | Mask Parameters::
      | 
      | Delay Depth (delay_depth): The length of the delay.
      | </pre>
  delay_lo : Subsystem  mask(SLR16 Delay){delay_depth=4}
      mask prompts: delay_depth "Delay Depth"
      mask help: A delay block that uses SLR16 elements for its storage.
      settings: AttributesFormatString=slr depth = 4
      mask Help:
      | <pre>
      | Description::
      | 
      | A delay block that uses SLR16 elements for its storage.
      | 
      | Mask Parameters::
      | 
      | Delay Depth (delay_depth): The length of the delay.
      | </pre>
  top_bit : xbsIndex_r3/Slice  mode=Upper Bit Location + Width  nbits=1  bit1=0  base1=MSB of Input  bit0=0  base0=LSB of Input  boolean_output=off  explicit_period=off  period=1  dbl_ovrd=off
  AloBlo : Outport
  AhiBhi : Outport  Port=2
  sync_out : Outport  Port=3
  wires:
  Delay/1 -> sync_out/1
  delay_lo/1(out) -> AloBlo/1
  Mux/1 -> delay_lo/1(in)
  delay_b/1(out) -> Mux/3, Mux1/2
  BloBhi/1 -> delay_b/1(in)
  Mux1/1 -> AhiBhi/1
  AloAhi/1 -> Mux1/3, Mux/2
  top_bit/1 -> Mux/1, Mux1/1
  Counter/1 -> top_bit/1
  sync_in/1 -> Delay/1, Counter/1
